simulink model "MBD1_LogicandBiwiseoperations"  (R2021a)
settings: Solver=FixedStepDiscrete  StartTime=0.0  StopTime=100  RelTol=1e-3
libraries: simulink x13
settings Model: Creator=Nour  LastModifiedBy=Nour
settings OptimizationCC: DefaultParameterBehavior=Inlined  EnhancedBackFolding=on  PassReuseOutputArgsAs=Individual arguments  ZeroExternalMemoryAtStartup=off  ZeroInternalMemoryAtStartup=off  OptimizeBlockOrder=speed  DifferentSizesBufferReuse=on  OptimizationCustomize=off  EfficientTunableParamExpr=on
settings DebuggingCC: ParameterTunabilityLossMsg=error
settings SFSimCC: MATLABDynamicMemAlloc=off
settings RTWCC: SystemTargetFile=ert.tlc  GenCodeOnly=on  TemplateMakefile=ert_default_tmf  GenerateReport=on  IncludeHyperlinkInReport=on  LaunchReport=on  GenerateTraceInfo=on
settings CodeAppCC: ForceParamTrailComments=on  IgnoreCustomStorageClasses=off  OperatorAnnotations=on  SimulinkDataObjDesc=on  SFDataObjDesc=on  InsertBlockDesc=on
settings ERTTargetCC: TargetLangStandard=C99 (ISO)  GenerateSampleERTMain=on  InlinedParameterPlacement=NonHierarchical  ERTCustomFileTemplate=example_file_process.tlc

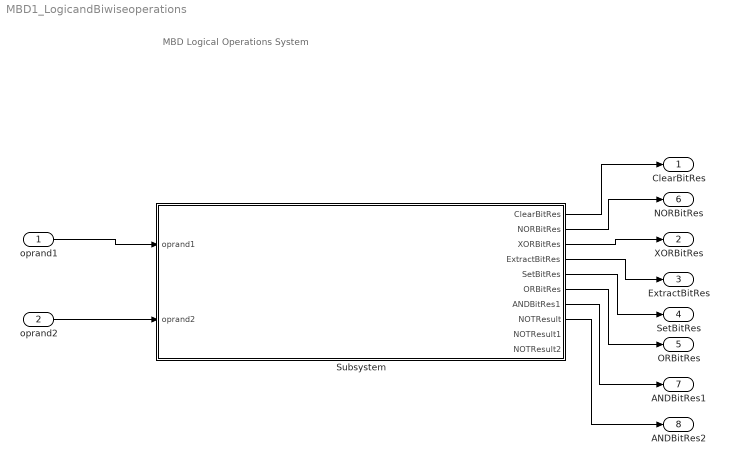
== system MBD1_LogicandBiwiseoperations ==
  note: MBD Logical Operations System
  oprand1 : Inport
  oprand2 : Inport  Port=2  OutDataTypeStr=uint8
  Subsystem : Subsystem
  ClearBitRes : Outport
  XORBitRes : Outport  Port=2
  ExtractBitRes : Outport  Port=3
  SetBitRes : Outport  Port=4
  ORBitRes : Outport  Port=5
  NORBitRes : Outport  Port=6
  ANDBitRes1 : Outport  Port=7
  ANDBitRes2 : Outport  Port=8
  wires:
  Subsystem/1(ClearBitRes) -> ClearBitRes/1
  Subsystem/6(ORBitRes) -> ORBitRes/1
  Subsystem/5(SetBitRes) -> SetBitRes/1
  Subsystem/4(ExtractBitRes) -> ExtractBitRes/1
  Subsystem/3(XORBitRes) -> XORBitRes/1
  Subsystem/2(NORBitRes) -> NORBitRes/1
  oprand2/1 -> Subsystem/2(oprand2)
  Subsystem/7(ANDBitRes1) -> ANDBitRes1/1
  oprand1/1 -> Subsystem/1(oprand1)
  Subsystem/8(NOTResult) -> ANDBitRes2/1

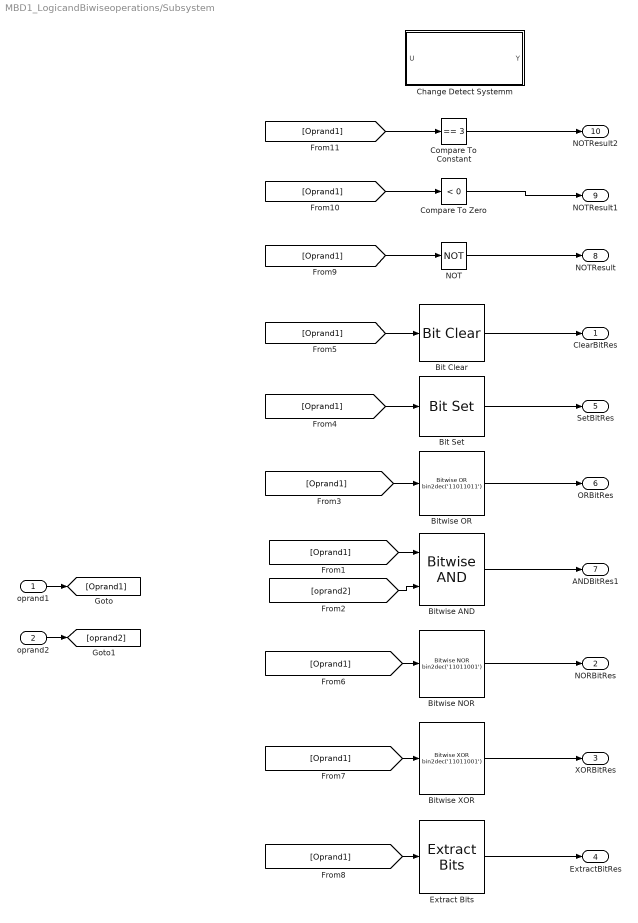
== system MBD1_LogicandBiwiseoperations/Subsystem ==
  oprand1 : Inport  OutDataTypeStr=uint8
  oprand2 : Inport  Port=2  OutDataTypeStr=uint8
  Bit Clear : simulink/Logic and Bit Operations/Bit Clear  iBit=0
      settings: SourceProductBaseCode=SL
  Bit Set : simulink/Logic and Bit Operations/Bit Set  iBit=0
      settings: SourceProductBaseCode=SL
  Bitwise AND : simulink/Logic and Bit Operations/Bitwise Operator  logicop=AND  UseBitMask=off  NumInputPorts=2  BitMask=bin2dec('11011001')  BitMaskRealWorld=Stored Integer
  Bitwise NOR : simulink/Logic and Bit Operations/Bitwise Operator  logicop=NOR  UseBitMask=on  BitMask=bin2dec('11011001')  BitMaskRealWorld=Stored Integer
  Bitwise OR : simulink/Logic and Bit Operations/Bitwise Operator  logicop=OR  UseBitMask=on  BitMask=bin2dec('11011011')  BitMaskRealWorld=Stored Integer
  Bitwise XOR : simulink/Logic and Bit Operations/Bitwise Operator  logicop=XOR  UseBitMask=on  BitMask=bin2dec('11011001')  BitMaskRealWorld=Stored Integer
  Change Detect Systemm : Subsystem
  Compare To Constant : simulink/Logic and Bit Operations/Compare To Constant  relop===  const=3  OutDataTypeStr=boolean
  Compare To Zero : simulink/Logic and Bit Operations/Compare To Zero  relop=<  OutDataTypeStr=boolean
  Extract Bits : simulink/Logic and Bit Operations/Extract Bits  bitsToExtract=Range of bits  numBits=8  bitIdxRange=[0 4]  outScalingMode=Preserve fixed-point scaling
  NOT : Logic  Operator=NOT  IconShape=distinctive  AllPortsSameDT=off  OutDataTypeStr=boolean
  ClearBitRes : Outport
  NORBitRes : Outport  Port=2
  XORBitRes : Outport  Port=3
  ExtractBitRes : Outport  Port=4
  SetBitRes : Outport  Port=5
  ORBitRes : Outport  Port=6
  ANDBitRes1 : Outport  Port=7
  NOTResult : Outport  Port=8
  NOTResult1 : Outport  Port=9  OutDataTypeStr=boolean
  NOTResult2 : Outport  Port=10  OutDataTypeStr=boolean
  wires:
  Extract Bits/1 -> ExtractBitRes/1
  Bit Set/1 -> SetBitRes/1
  [Oprand1] -> Bit Set/1
  Bitwise NOR/1 -> NORBitRes/1
  Bitwise OR/1 -> ORBitRes/1
  oprand1/1 -> [Oprand1]
  [Oprand1] -> Bitwise NOR/1
  Bitwise XOR/1 -> XORBitRes/1
  [Oprand1] -> Bit Clear/1
  [Oprand1] -> Bitwise OR/1
  [Oprand1] -> Bitwise XOR/1
  [Oprand1] -> Extract Bits/1
  Bit Clear/1 -> ClearBitRes/1
  Bitwise AND/1 -> ANDBitRes1/1
  [Oprand1] -> Bitwise AND/1
  [oprand2] -> Bitwise AND/2
  oprand2/1 -> [oprand2]
  [Oprand1] -> NOT/1
  NOT/1 -> NOTResult/1
  [Oprand1] -> Compare To Zero/1
  [Oprand1] -> Compare To Constant/1
  Compare To Zero/1 -> NOTResult1/1
  Compare To Constant/1 -> NOTResult2/1

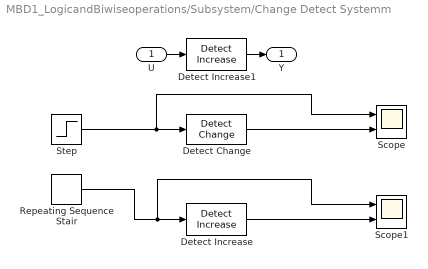
== system MBD1_LogicandBiwiseoperations/Subsystem/Change Detect Systemm ==
  U : Inport
  Detect Change : simulink/Logic and Bit Operations/Detect Change  vinit=0  OutDataTypeStr=boolean
  Detect Increase : simulink/Logic and Bit Operations/Detect Increase  vinit=0.0  OutDataTypeStr=boolean
  Detect Increase1 : simulink/Logic and Bit Operations/Detect Increase  vinit=0.0  OutDataTypeStr=boolean
  Repeating Sequence Stair : simulink/Sources/Repeating Sequence Stair  OutValues=[3 1 4 2 1].'  tsamp=-1  OutMin=[]  OutMax=[]  OutDataTypeStr=double  OutputDataTypeScalingMode=double  OutDataType=fixdt(0,8)  ConRadixGroup=Best Precision: Vector-wise  OutScaling=2^-12
  Scope : Scope  NumInputPorts=2
  Scope1 : Scope  NumInputPorts=2
  Step : Step  Time=2
  Y : Outport
  wires:
  Repeating Sequence Stair/1 -> Scope1/1, Detect Increase/1
  Step/1 -> Scope/1, Detect Change/1
  Detect Increase1/1 -> Y/1
  Detect Change/1 -> Scope/2
  U/1 -> Detect Increase1/1
  Detect Increase/1 -> Scope1/2
